simulink model "SWC_FDC_type"  (R2021b)
settings: Solver=FixedStepDiscrete  StartTime=0.0  StopTime=10.0  FixedStep=0.001  RelTol=1e-3
values from neighbouring files (symbols this model uses):
  C_TASK_5MS_S = (	C_TICK_TIME_S      	)    [vcu_local_hdr.m]
  DID_VCUKey = uint16(0x0202)    [vcu_local_hdr.m]
  DID_XWD = uint16(513)    [vcu_local_hdr.m]
  DIDLen_DKCKey = uint16(8)    [vcu_local_hdr.m]
  DIDLen_FoxPiBattSta = uint16(4)    [vcu_local_hdr.m]
  DIDLen_FoxPiBrakeSta = uint16(13)    [vcu_local_hdr.m]
  DIDLen_FoxPiButtonSta = uint16(2)    [vcu_local_hdr.m]
  DIDLen_FoxPiCtrlEnSw = uint16(1)    [vcu_local_hdr.m]
  DIDLen_FoxPiDrivingCtrl = uint16(21)    [vcu_local_hdr.m]
  DIDLen_FoxPiEPSSta = uint16(11)    [vcu_local_hdr.m]
  DIDLen_FoxPiLampCtrl = uint16(6)    [vcu_local_hdr.m]
  DIDLen_FoxPiLampSta = uint16(2)    [vcu_local_hdr.m]
  DIDLen_FoxPiMotionSta = uint16(13)    [vcu_local_hdr.m]
  DIDLen_FoxPiMotorSta = uint16(11)    [vcu_local_hdr.m]
  DIDLen_FoxPiPedalPos = uint16(3)    [vcu_local_hdr.m]
  DIDLen_FoxPiPTGUSSSw = uint16(1)    [vcu_local_hdr.m]
  DIDLen_FoxPiShifterAllow = uint16(3)    [vcu_local_hdr.m]
  DIDLen_FoxPiSwSta = uint16(2)    [vcu_local_hdr.m]
  DIDLen_FoxPiTPMSSta = uint16(13)    [vcu_local_hdr.m]
  DIDLen_FoxPiUSSDist = uint16(20)    [vcu_local_hdr.m]
  DIDLen_FoxPiUSSFaultSta = uint16(2)    [vcu_local_hdr.m]
  DIDLen_FoxPiWheelSpd = uint16(16)    [vcu_local_hdr.m]
  DIDNum_DKCKey = uint16(0x0202)    [vcu_local_hdr.m]
  DIDNum_FoxPiBattSta = uint16(0x100D)    [vcu_local_hdr.m]
  DIDNum_FoxPiBrakeSta = uint16(0x1003)    [vcu_local_hdr.m]
  DIDNum_FoxPiButtonSta = uint16(0x1006)    [vcu_local_hdr.m]
  DIDNum_FoxPiCtrlEnSw = uint16(0x1012)    [vcu_local_hdr.m]
  DIDNum_FoxPiDrivingCtrl = uint16(0x1001)    [vcu_local_hdr.m]
  DIDNum_FoxPiEPSSta = uint16(0x1005)    [vcu_local_hdr.m]
  DIDNum_FoxPiLampCtrl = uint16(0x100C)    [vcu_local_hdr.m]
  DIDNum_FoxPiLampSta = uint16(0x100B)    [vcu_local_hdr.m]
  DIDNum_FoxPiMotionSta = uint16(0x1002)    [vcu_local_hdr.m]
  DIDNum_FoxPiMotorSta = uint16(0x1010)    [vcu_local_hdr.m]
  DIDNum_FoxPiPedalPos = uint16(0x100F)    [vcu_local_hdr.m]
  DIDNum_FoxPiPTGUSSSw = uint16(0x1009)    [vcu_local_hdr.m]
  DIDNum_FoxPiShifterAllow = uint16(0x1011)    [vcu_local_hdr.m]
  DIDNum_FoxPiSwSta = uint16(0x100A)    [vcu_local_hdr.m]
  DIDNum_FoxPiTPMSSta = uint16(0x100E)    [vcu_local_hdr.m]
  DIDNum_FoxPiUSSDist = uint16(0x1007)    [vcu_local_hdr.m]
  DIDNum_FoxPiUSSFaultSta = uint16(0x1008)    [vcu_local_hdr.m]
  DIDNum_FoxPiWheelSpd = uint16(0x1004)    [vcu_local_hdr.m]
  DIDVCUKeyLength = uint16(8)    [vcu_local_hdr.m]
  DTC_10020B = Simulink.Parameter    [DTC_Constant_Definition.m]
  DTC_10020C = Simulink.Parameter    [DTC_Constant_Definition.m]
  DTC_10020D = Simulink.Parameter    [DTC_Constant_Definition.m]
  DTC_10020E = Simulink.Parameter    [DTC_Constant_Definition.m]
  DTC_100210 = Simulink.Parameter    [DTC_Constant_Definition.m]
  DTC_100211 = Simulink.Parameter    [DTC_Constant_Definition.m]
  DTC_100212 = Simulink.Parameter    [DTC_Constant_Definition.m]
  DTC_100213 = Simulink.Parameter    [DTC_Constant_Definition.m]
  DTC_100214 = Simulink.Parameter    [DTC_Constant_Definition.m]
  DTC_100215 = Simulink.Parameter    [DTC_Constant_Definition.m]
  DTC_100216 = Simulink.Parameter    [DTC_Constant_Definition.m]
  DTC_100217 = Simulink.Parameter    [DTC_Constant_Definition.m]
  DTC_100218 = Simulink.Parameter    [DTC_Constant_Definition.m]
  DTC_100219 = Simulink.Parameter    [DTC_Constant_Definition.m]
  DTC_10021A = Simulink.Parameter    [DTC_Constant_Definition.m]
  DTC_10021B = Simulink.Parameter    [DTC_Constant_Definition.m]
  DTC_10021C = Simulink.Parameter    [DTC_Constant_Definition.m]
  DTC_10021D = Simulink.Parameter    [DTC_Constant_Definition.m]
  DTC_10021E = Simulink.Parameter    [DTC_Constant_Definition.m]
  DTC_100220 = Simulink.Parameter    [DTC_Constant_Definition.m]
  DTC_100221 = Simulink.Parameter    [DTC_Constant_Definition.m]
  DTC_100223 = Simulink.Parameter    [DTC_Constant_Definition.m]
  DTC_100224 = Simulink.Parameter    [DTC_Constant_Definition.m]
  DTC_100225 = Simulink.Parameter    [DTC_Constant_Definition.m]
  DTC_100226 = Simulink.Parameter    [DTC_Constant_Definition.m]
  DTC_100227 = Simulink.Parameter    [DTC_Constant_Definition.m]
  DTC_100242 = Simulink.Parameter    [DTC_Constant_Definition.m]
  DTC_100243 = Simulink.Parameter    [DTC_Constant_Definition.m]
  DTC_100244 = Simulink.Parameter    [DTC_Constant_Definition.m]
  DTC_100247 = Simulink.Parameter    [DTC_Constant_Definition.m]
  DTC_100248 = Simulink.Parameter    [DTC_Constant_Definition.m]
  DTC_100249 = Simulink.Parameter    [DTC_Constant_Definition.m]
  DTC_100250 = Simulink.Parameter    [DTC_Constant_Definition.m]
  DTC_100251 = Simulink.Parameter    [DTC_Constant_Definition.m]
  DTC_100252 = Simulink.Parameter    [DTC_Constant_Definition.m]
  DTC_100A10 = Simulink.Parameter    [DTC_Constant_Definition.m]
  DTC_100A12 = Simulink.Parameter    [DTC_Constant_Definition.m]
  DTC_100A16 = Simulink.Parameter    [DTC_Constant_Definition.m]
  DTC_100A17 = Simulink.Parameter    [DTC_Constant_Definition.m]
  DTC_100A18 = Simulink.Parameter    [DTC_Constant_Definition.m]
  DTC_100A19 = Simulink.Parameter    [DTC_Constant_Definition.m]
  DTC_500B01 = Simulink.Parameter    [DTC_Constant_Definition.m]
  DTC_500B02 = Simulink.Parameter    [DTC_Constant_Definition.m]
  DTC_500B03 = Simulink.Parameter    [DTC_Constant_Definition.m]
  DTC_500B04 = Simulink.Parameter    [DTC_Constant_Definition.m]
  DTC_500B05 = Simulink.Parameter    [DTC_Constant_Definition.m]
  DTC_500B06 = Simulink.Parameter    [DTC_Constant_Definition.m]
  DTC_500B07 = Simulink.Parameter    [DTC_Constant_Definition.m]
  DTC_500B08 = Simulink.Parameter    [DTC_Constant_Definition.m]
  DTC_500B09 = Simulink.Parameter    [DTC_Constant_Definition.m]
  DTC_500B0A = Simulink.Parameter    [DTC_Constant_Definition.m]
  DTC_500B0B = Simulink.Parameter    [DTC_Constant_Definition.m]
  DTC_500B0C = Simulink.Parameter    [DTC_Constant_Definition.m]
  DTC_500B0D = Simulink.Parameter    [DTC_Constant_Definition.m]
  DTC_500B0E = Simulink.Parameter    [DTC_Constant_Definition.m]
  DTC_500B0F = Simulink.Parameter    [DTC_Constant_Definition.m]
  DTC_500B10 = Simulink.Parameter    [DTC_Constant_Definition.m]
  DTC_90021F = Simulink.Parameter    [DTC_Constant_Definition.m]
  DTC_90022F = Simulink.Parameter    [DTC_Constant_Definition.m]
  DTC_900253 = Simulink.Parameter    [DTC_Constant_Definition.m]
  DTC_900254 = Simulink.Parameter    [DTC_Constant_Definition.m]
  DTC_900301 = Simulink.Parameter    [DTC_Constant_Definition.m]
  DTC_900302 = Simulink.Parameter    [DTC_Constant_Definition.m]
  DTC_900303 = Simulink.Parameter    [DTC_Constant_Definition.m]
  DTC_900304 = Simulink.Parameter    [DTC_Constant_Definition.m]
  DTC_900305 = Simulink.Parameter    [DTC_Constant_Definition.m]
  DTC_900909 = Simulink.Parameter    [DTC_Constant_Definition.m]
  DTC_90090A = Simulink.Parameter    [DTC_Constant_Definition.m]
  DTC_90090B = Simulink.Parameter    [DTC_Constant_Definition.m]
  DTC_90090C = Simulink.Parameter    [DTC_Constant_Definition.m]
  DTC_90090D = Simulink.Parameter    [DTC_Constant_Definition.m]
  DTC_90090E = Simulink.Parameter    [DTC_Constant_Definition.m]
  DTC_90090F = Simulink.Parameter    [DTC_Constant_Definition.m]
  DTC_900910 = Simulink.Parameter    [DTC_Constant_Definition.m]
  DTC_900911 = Simulink.Parameter    [DTC_Constant_Definition.m]
  DTC_900912 = Simulink.Parameter    [DTC_Constant_Definition.m]
  DTC_900913 = Simulink.Parameter    [DTC_Constant_Definition.m]
  DTC_900914 = Simulink.Parameter    [DTC_Constant_Definition.m]
  ... (+54 more)
undefined symbols (not defined in the file or in its folder): f32_ApsOutVehSpdSig, KHAL_CANBusOffDebounce_cnt, KHAL_CANBusOffDebounce_s, KHAL_DKCDecryptEnable_flg_ovrdflg, KHAL_DKCDecryptEnable_flg_ovrdval, KHAL_RandomNumberY1_enum, KHAL_RandomNumberY2_enum, KHAL_RandomNumberY_ovrdflg, KHAL_TPMSRESBUTT_flg_ovrdflg, KHAL_TPMSRESBUTT_flg_ovrdval, KINP_ReadVinCode_flg, P_boolean, R_DIDWriteCDD_CSOP_DIDSet_DKCKey, R_DIDWriteCDD_CSOP_DIDSet_FoxPiBattSta, R_DIDWriteCDD_CSOP_DIDSet_FoxPiBrakeSta, R_DIDWriteCDD_CSOP_DIDSet_FoxPiButtonSta, R_DIDWriteCDD_CSOP_DIDSet_FoxPiCtrlEnSw, R_DIDWriteCDD_CSOP_DIDSet_FoxPiDrivingCtrl, R_DIDWriteCDD_CSOP_DIDSet_FoxPiEPSSta, R_DIDWriteCDD_CSOP_DIDSet_FoxPiLampCtrl, R_DIDWriteCDD_CSOP_DIDSet_FoxPiLampSta, R_DIDWriteCDD_CSOP_DIDSet_FoxPiMotionSta, R_DIDWriteCDD_CSOP_DIDSet_FoxPiMotorSta, R_DIDWriteCDD_CSOP_DIDSet_FoxPiPedalPos, R_DIDWriteCDD_CSOP_DIDSet_FoxPiPTGUSSSw, R_DIDWriteCDD_CSOP_DIDSet_FoxPiShifterAllow, R_DIDWriteCDD_CSOP_DIDSet_FoxPiSwSta, R_DIDWriteCDD_CSOP_DIDSet_FoxPiTPMSSta, R_DIDWriteCDD_CSOP_DIDSet_FoxPiUSSDist, R_DIDWriteCDD_CSOP_DIDSet_FoxPiUSSFaultSta, R_DIDWriteCDD_CSOP_DIDSet_FoxPiWheelSpd, R_E2E_CAN3_VCU1_CSOP_Write_CAN3_VCU1, R_E2E_CAN3_VCU1_toNIDEC_CSOP_Write_CAN3_VCU1_toNIDEC, R_E2E_CAN4_VCU1_CSOP_Write_CAN4_VCU1, R_FDCCDD_Inner_CSOP_FDC_AppCallSleep, R_HALIN_IMU_CSOP_IMUSetSta, R_HALINCDD_CSOP_PAS_Handler, R_HALINCDD_CSOP_ResetPedalZeroPosDone, R_HALINCDD_CSOP_TPMSSensorIDRegSetResults, R_HALINCDD_CSOP_UDS_Main, R_HALOUT_APS_CSOP_ApsOutput, R_HALOUTCDD_CSOP_AppNmStateReq, R_HALOUTCDD_CSOP_IVIReset, R_HALOUTCDD_CSOP_SetAcoreRebootCmdACK, R_HALOUTCDD_CSOP_SetSysPwrStat ... (+80)
libraries: FVT_lib x447, simulink x289, hcu_lib x19, hdlsllib x9, app x1, halin x1, halout x1, matrix_library x1, inp x1, outp x1
(part 12 of 15)

== system SWC_FDC_type/run_SWC_FDC_RxTx_5ms_sys/Halin_CDD/Halin_SYS/FlashMFSWTri_Verify ==
  In1 : Inport
  Compare To Constant : simulink/Logic and Bit Operations/Compare To Constant  relop=>  const=1  OutDataTypeStr=boolean
  Compare To Constant1 : simulink/Logic and Bit Operations/Compare To Constant  relop=<  const=0  OutDataTypeStr=boolean
  Constant : Constant  Value=ZERO_INT
  Logical Operator : Logic  Operator=OR  AllPortsSameDT=off  OutDataTypeStr=boolean
  Switch : Switch  Criteria=u2 > Threshold
  Out1 : Outport
  wires:
  Compare To Constant1/1 -> Logical Operator/2
  Compare To Constant/1 -> Logical Operator/1
  Logical Operator/1 -> Switch/2
  Switch/1 -> Out1/1
  Constant/1 -> Switch/1
  In1/1 -> Compare To Constant/1, Compare To Constant1/1, Switch/3

== system SWC_FDC_type/run_SWC_FDC_RxTx_5ms_sys/Halin_CDD/Halin_SYS/FlashMirrorFlodPos_Verify ==
  In1 : Inport
  Compare To Constant : simulink/Logic and Bit Operations/Compare To Constant  relop=>  const=1  OutDataTypeStr=boolean
  Compare To Constant1 : simulink/Logic and Bit Operations/Compare To Constant  relop=<  const=0  OutDataTypeStr=boolean
  Constant : Constant  Value=ZERO_INT
  Logical Operator : Logic  Operator=OR  AllPortsSameDT=off  OutDataTypeStr=boolean
  Switch : Switch  Criteria=u2 > Threshold
  Out1 : Outport
  wires:
  In1/1 -> Switch/3, Compare To Constant1/1, Compare To Constant/1
  Constant/1 -> Switch/1
  Switch/1 -> Out1/1
  Logical Operator/1 -> Switch/2
  Compare To Constant/1 -> Logical Operator/1
  Compare To Constant1/1 -> Logical Operator/2

== system SWC_FDC_type/run_SWC_FDC_RxTx_5ms_sys/Halin_CDD/Halin_SYS/FlashRecAutoFlg_Verify ==
  In1 : Inport
  Compare To Constant : simulink/Logic and Bit Operations/Compare To Constant  relop=>  const=1  OutDataTypeStr=boolean
  Compare To Constant1 : simulink/Logic and Bit Operations/Compare To Constant  relop=<  const=0  OutDataTypeStr=boolean
  Constant : Constant  Value=ZERO_INT
  Logical Operator : Logic  Operator=OR  AllPortsSameDT=off  OutDataTypeStr=boolean
  Switch : Switch  Criteria=u2 > Threshold
  Out1 : Outport
  wires:
  In1/1 -> Switch/3, Compare To Constant1/1, Compare To Constant/1
  Constant/1 -> Switch/1
  Switch/1 -> Out1/1
  Logical Operator/1 -> Switch/2
  Compare To Constant/1 -> Logical Operator/1
  Compare To Constant1/1 -> Logical Operator/2

== system SWC_FDC_type/run_SWC_FDC_RxTx_5ms_sys/Halin_CDD/Halin_SYS/FlashWiperFixMode_Verify ==
  In1 : Inport
  Compare To Constant : simulink/Logic and Bit Operations/Compare To Constant  relop=>  const=1  OutDataTypeStr=boolean
  Compare To Constant1 : simulink/Logic and Bit Operations/Compare To Constant  relop=<  const=0  OutDataTypeStr=boolean
  Constant : Constant  Value=ZERO_INT
  Logical Operator : Logic  Operator=OR  AllPortsSameDT=off  OutDataTypeStr=boolean
  Switch : Switch  Criteria=u2 > Threshold
  Out1 : Outport
  wires:
  Compare To Constant1/1 -> Logical Operator/2
  Compare To Constant/1 -> Logical Operator/1
  Logical Operator/1 -> Switch/2
  Switch/1 -> Out1/1
  Constant/1 -> Switch/1
  In1/1 -> Compare To Constant/1, Compare To Constant1/1, Switch/3

== system SWC_FDC_type/run_SWC_FDC_RxTx_5ms_sys/Halin_CDD/Halin_SYS/Flashfdefog_Verify ==
  In1 : Inport
  Compare To Constant : simulink/Logic and Bit Operations/Compare To Constant  relop=>  const=1  OutDataTypeStr=boolean
  Compare To Constant1 : simulink/Logic and Bit Operations/Compare To Constant  relop=<  const=0  OutDataTypeStr=boolean
  Constant : Constant  Value=ZERO_INT
  Logical Operator : Logic  Operator=OR  AllPortsSameDT=off  OutDataTypeStr=boolean
  Switch : Switch  Criteria=u2 > Threshold
  Out1 : Outport
  wires:
  In1/1 -> Switch/3, Compare To Constant1/1, Compare To Constant/1
  Constant/1 -> Switch/1
  Switch/1 -> Out1/1
  Logical Operator/1 -> Switch/2
  Compare To Constant/1 -> Logical Operator/1
  Compare To Constant1/1 -> Logical Operator/2

== system SWC_FDC_type/run_SWC_FDC_RxTx_5ms_sys/Halin_CDD/Halin_SYS/FlashsigRecircSt_Verify ==
  In1 : Inport
  Compare To Constant : simulink/Logic and Bit Operations/Compare To Constant  relop=>  const=1  OutDataTypeStr=boolean
  Compare To Constant1 : simulink/Logic and Bit Operations/Compare To Constant  relop=<  const=0  OutDataTypeStr=boolean
  Constant : Constant  Value=ZERO_INT
  Logical Operator : Logic  Operator=OR  AllPortsSameDT=off  OutDataTypeStr=boolean
  Switch : Switch  Criteria=u2 > Threshold
  Out1 : Outport
  wires:
  Compare To Constant1/1 -> Logical Operator/2
  Compare To Constant/1 -> Logical Operator/1
  Logical Operator/1 -> Switch/2
  Switch/1 -> Out1/1
  Constant/1 -> Switch/1
  In1/1 -> Compare To Constant/1, Compare To Constant1/1, Switch/3

== system SWC_FDC_type/run_SWC_FDC_RxTx_5ms_sys/Halin_CDD/Halin_SYS/FlashsigSetTempZon1St_Verify ==
  In1 : Inport
  Compare To Constant : simulink/Logic and Bit Operations/Compare To Constant  relop=>  const=32  OutDataTypeStr=boolean
  Compare To Constant1 : simulink/Logic and Bit Operations/Compare To Constant  relop=<  const=17  OutDataTypeStr=boolean
  Constant : Constant  Value=25
  Logical Operator : Logic  Operator=OR  AllPortsSameDT=off  OutDataTypeStr=boolean
  Switch : Switch  Criteria=u2 > Threshold
  Out1 : Outport
  wires:
  In1/1 -> Switch/3, Compare To Constant1/1, Compare To Constant/1
  Constant/1 -> Switch/1
  Switch/1 -> Out1/1
  Logical Operator/1 -> Switch/2
  Compare To Constant/1 -> Logical Operator/1
  Compare To Constant1/1 -> Logical Operator/2

== system SWC_FDC_type/run_SWC_FDC_RxTx_5ms_sys/Halin_CDD/Halin_SYS/FlashsigSetTempZon2StM_Verify ==
  In1 : Inport
  Compare To Constant : simulink/Logic and Bit Operations/Compare To Constant  relop=>  const=32  OutDataTypeStr=boolean
  Compare To Constant1 : simulink/Logic and Bit Operations/Compare To Constant  relop=<  const=17  OutDataTypeStr=boolean
  Constant : Constant  Value=25
  Logical Operator : Logic  Operator=OR  AllPortsSameDT=off  OutDataTypeStr=boolean
  Switch : Switch  Criteria=u2 > Threshold
  Out1 : Outport
  wires:
  Compare To Constant1/1 -> Logical Operator/2
  Compare To Constant/1 -> Logical Operator/1
  Logical Operator/1 -> Switch/2
  Switch/1 -> Out1/1
  Constant/1 -> Switch/1
  In1/1 -> Compare To Constant/1, Compare To Constant1/1, Switch/3

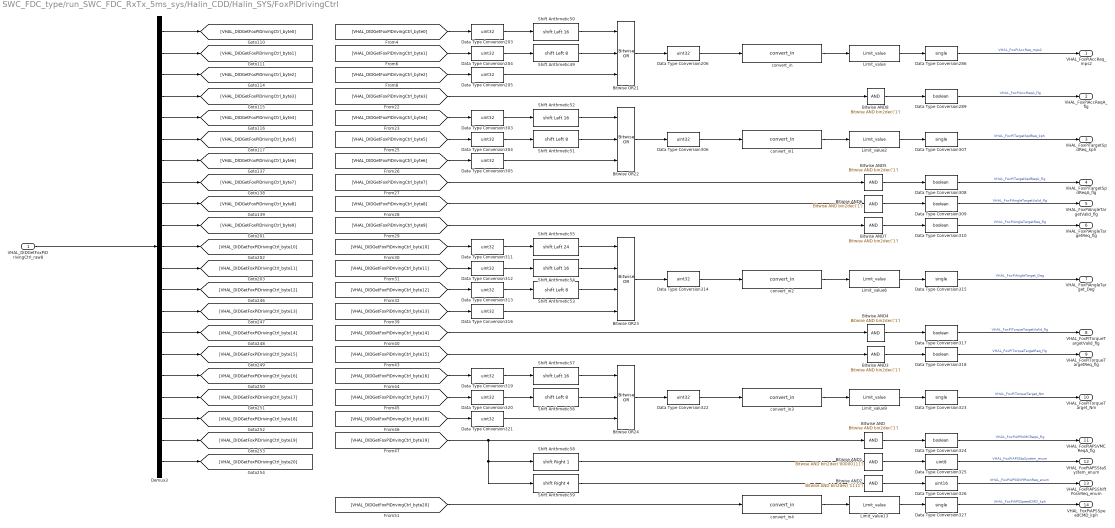
== system SWC_FDC_type/run_SWC_FDC_RxTx_5ms_sys/Halin_CDD/Halin_SYS/FoxPiDrivingCtrl ==
  VHAL_DIDGetFoxPiDrivingCtrl_raw8 : Inport
  Bitwise AND{,3..8} (7 alike) : simulink/Logic and Bit Operations/Bitwise Operator  logicop=AND  UseBitMask=on  BitMask=bin2dec('1')  BitMaskRealWorld=Stored Integer
  Bitwise AND1 : simulink/Logic and Bit Operations/Bitwise Operator  logicop=AND  UseBitMask=on  BitMask=bin2dec('00000111')  BitMaskRealWorld=Stored Integer
  Bitwise AND2 : simulink/Logic and Bit Operations/Bitwise Operator  logicop=AND  UseBitMask=on  BitMask=bin2dec('1111')  BitMaskRealWorld=Stored Integer
  Bitwise OR21 : simulink/Logic and Bit Operations/Bitwise Operator  logicop=OR  UseBitMask=off  NumInputPorts=3  BitMask=bin2dec('00000000000000000000')  BitMaskRealWorld=Stored Integer
  Bitwise OR22 : simulink/Logic and Bit Operations/Bitwise Operator  logicop=OR  UseBitMask=off  NumInputPorts=3  BitMask=bin2dec('00000000000000000000')  BitMaskRealWorld=Stored Integer
  Bitwise OR23 : simulink/Logic and Bit Operations/Bitwise Operator  logicop=OR  UseBitMask=off  NumInputPorts=4  BitMask=bin2dec('00000000000000000000')  BitMaskRealWorld=Stored Integer
  Bitwise OR24 : simulink/Logic and Bit Operations/Bitwise Operator  logicop=OR  UseBitMask=off  NumInputPorts=3  BitMask=bin2dec('00000000000000000000')  BitMaskRealWorld=Stored Integer
  Data Type Conversion{203..206,303..306,311..314,316,319..322} (17 alike) : DataTypeConversion  OutDataTypeStr=uint32
  Data Type Conversion{286,307,315,323,327} (5 alike) : DataTypeConversion  OutDataTypeStr=single
  Data Type Conversion{289,308..310,317..318,324} (7 alike) : DataTypeConversion  OutDataTypeStr=boolean
  Data Type Conversion325 : DataTypeConversion  OutDataTypeStr=uint8
  Data Type Conversion326 : DataTypeConversion  OutDataTypeStr=uint16
  Demux3 : Demux  Outputs=21
  Limit_value : FVT_lib/hal/Limit_value  Upper_limit=10.55  Lower_limit=-15
  Limit_value13 : FVT_lib/hal/Limit_value  Upper_limit=20  Lower_limit=0
  Limit_value2 : FVT_lib/hal/Limit_value  Upper_limit=255.875  Lower_limit=0
  Limit_value6 : FVT_lib/hal/Limit_value  Upper_limit=900  Lower_limit=-900
  Limit_value9 : FVT_lib/hal/Limit_value  Upper_limit=10  Lower_limit=-10
  Shift Arithmetic{49,51,53,56} (4 alike) : ArithShift  BitShiftNumber=8  BitShiftDirection=Left
  Shift Arithmetic{50,52,54,57} (4 alike) : ArithShift  BitShiftNumber=16  BitShiftDirection=Left
  Shift Arithmetic55 : ArithShift  BitShiftNumber=24  BitShiftDirection=Left
  Shift Arithmetic58 : ArithShift  BitShiftNumber=1  BitShiftDirection=Right
  Shift Arithmetic59 : ArithShift  BitShiftNumber=4  BitShiftDirection=Right
  convert_in : FVT_lib/hal/convert_in  gain=0.05  offset=-15
  convert_in1 : FVT_lib/hal/convert_in  gain=0.125  offset=0
  convert_in2 : FVT_lib/hal/convert_in  gain=0.1  offset=-900
  convert_in3 : FVT_lib/hal/convert_in  gain=0.01  offset=-10
  convert_in4 : FVT_lib/hal/convert_in  gain=0.125  offset=0
  VHAL_FoxPiAccReq_mps2 : Outport
  VHAL_FoxPiAccReqA_flg : Outport  Port=2
  VHAL_FoxPiTargetSpdReq_kph : Outport  Port=3
  VHAL_FoxPiTargetSpdReqA_flg : Outport  Port=4
  VHAL_FoxPiAngleTargetValid_flg : Outport  Port=5
  VHAL_FoxPiAngleTargetReq_flg : Outport  Port=6
  VHAL_FoxPiAngleTarget_Deg : Outport  Port=7
  VHAL_FoxPiTorqueTargetValid_flg : Outport  Port=8
  VHAL_FoxPiTorqueTargetReq_flg : Outport  Port=9
  VHAL_FoxPiTorqueTarget_Nm : Outport  Port=10
  VHAL_FoxPiAPSVMCReqA_flg : Outport  Port=11
  VHAL_FoxPiAPSStaSystem_enum : Outport  Port=12
  VHAL_FoxPiAPSShiftPosnReq_enum : Outport  Port=13
  VHAL_FoxPiAPSSpeedCMD_kph : Outport  Port=14
  wires:
  [VHAL_DIDGetFoxPiDrivingCtrl_byte10] -> Data Type Conversion311/1
  [VHAL_DIDGetFoxPiDrivingCtrl_byte20] -> convert_in4/1
  convert_in3/1 -> Limit_value9/1
  [VHAL_DIDGetFoxPiDrivingCtrl_byte14] -> Bitwise AND4/1
  Demux3/14 -> [VHAL_DIDGetFoxPiDrivingCtrl_byte13]
  Data Type Conversion322/1 -> convert_in3/1
  [VHAL_DIDGetFoxPiDrivingCtrl_byte1] -> Data Type Conversion204/1
  [VHAL_DIDGetFoxPiDrivingCtrl_byte19] -> Shift Arithmetic59/1, Shift Arithmetic58/1, Bitwise AND/1
  Data Type Conversion309/1 -> VHAL_FoxPiAngleTargetValid_flg/1  "VHAL_FoxPiAngleTargetValid_flg"
  Data Type Conversion324/1 -> VHAL_FoxPiAPSVMCReqA_flg/1  "VHAL_FoxPiAPSVMCReqA_flg"
  Demux3/4 -> [VHAL_DIDGetFoxPiDrivingCtrl_byte3]
  [VHAL_DIDGetFoxPiDrivingCtrl_byte7] -> Bitwise AND5/1
  [VHAL_DIDGetFoxPiDrivingCtrl_byte8] -> Bitwise AND6/1
  [VHAL_DIDGetFoxPiDrivingCtrl_byte11] -> Data Type Conversion312/1
  [VHAL_DIDGetFoxPiDrivingCtrl_byte5] -> Data Type Conversion304/1
  Bitwise OR24/1 -> Data Type Conversion322/1
  Data Type Conversion325/1 -> VHAL_FoxPiAPSStaSystem_enum/1  "VHAL_FoxPiAPSStaSystem_enum"
  [VHAL_DIDGetFoxPiDrivingCtrl_byte17] -> Data Type Conversion320/1
  Data Type Conversion314/1 -> convert_in2/1
  [VHAL_DIDGetFoxPiDrivingCtrl_byte16] -> Data Type Conversion319/1
  Bitwise OR22/1 -> Data Type Conversion306/1
  Shift Arithmetic59/1 -> Bitwise AND2/1
  Demux3/2 -> [VHAL_DIDGetFoxPiDrivingCtrl_byte1]
  [VHAL_DIDGetFoxPiDrivingCtrl_byte12] -> Data Type Conversion313/1
  [VHAL_DIDGetFoxPiDrivingCtrl_byte2] -> Data Type Conversion205/1
  Data Type Conversion306/1 -> convert_in1/1
  [VHAL_DIDGetFoxPiDrivingCtrl_byte4] -> Data Type Conversion303/1
  Data Type Conversion307/1 -> VHAL_FoxPiTargetSpdReq_kph/1  "VHAL_FoxPiTargetSpdReq_kph"
  Data Type Conversion326/1 -> VHAL_FoxPiAPSShiftPosnReq_enum/1  "VHAL_FoxPiAPSShiftPosnReq_enum"
  Data Type Conversion304/1 -> Shift Arithmetic51/1
  Demux3/1 -> [VHAL_DIDGetFoxPiDrivingCtrl_byte0]
  convert_in4/1 -> Limit_value13/1
  Data Type Conversion323/1 -> VHAL_FoxPiTorqueTarget_Nm/1  "VHAL_FoxPiTorqueTarget_Nm"
  [VHAL_DIDGetFoxPiDrivingCtrl_byte9] -> Bitwise AND7/1
  [VHAL_DIDGetFoxPiDrivingCtrl_byte13] -> Data Type Conversion316/1
  Demux3/11 -> [VHAL_DIDGetFoxPiDrivingCtrl_byte10]
  Bitwise OR21/1 -> Data Type Conversion206/1
  convert_in2/1 -> Limit_value6/1
  [VHAL_DIDGetFoxPiDrivingCtrl_byte18] -> Data Type Conversion321/1
  Demux3/3 -> [VHAL_DIDGetFoxPiDrivingCtrl_byte2]
  Bitwise OR23/1 -> Data Type Conversion314/1
  Data Type Conversion206/1 -> convert_in/1
  [VHAL_DIDGetFoxPiDrivingCtrl_byte6] -> Data Type Conversion305/1
  [VHAL_DIDGetFoxPiDrivingCtrl_byte15] -> Bitwise AND3/1
  convert_in1/1 -> Limit_value2/1
  [VHAL_DIDGetFoxPiDrivingCtrl_byte0] -> Data Type Conversion203/1
  Shift Arithmetic58/1 -> Bitwise AND1/1
  Demux3/7 -> [VHAL_DIDGetFoxPiDrivingCtrl_byte6]
  Demux3/8 -> [VHAL_DIDGetFoxPiDrivingCtrl_byte7]
  Demux3/5 -> [VHAL_DIDGetFoxPiDrivingCtrl_byte4]
  Demux3/6 -> [VHAL_DIDGetFoxPiDrivingCtrl_byte5]
  Demux3/10 -> [VHAL_DIDGetFoxPiDrivingCtrl_byte9]
  Demux3/12 -> [VHAL_DIDGetFoxPiDrivingCtrl_byte11]
  Demux3/9 -> [VHAL_DIDGetFoxPiDrivingCtrl_byte8]
  Demux3/13 -> [VHAL_DIDGetFoxPiDrivingCtrl_byte12]
  Demux3/21 -> [VHAL_DIDGetFoxPiDrivingCtrl_byte20]
  Demux3/15 -> [VHAL_DIDGetFoxPiDrivingCtrl_byte14]
  Demux3/16 -> [VHAL_DIDGetFoxPiDrivingCtrl_byte15]
  Data Type Conversion317/1 -> VHAL_FoxPiTorqueTargetValid_flg/1  "VHAL_FoxPiTorqueTargetValid_flg"
  Demux3/17 -> [VHAL_DIDGetFoxPiDrivingCtrl_byte16]
  Demux3/20 -> [VHAL_DIDGetFoxPiDrivingCtrl_byte19]
  Demux3/18 -> [VHAL_DIDGetFoxPiDrivingCtrl_byte17]
  Demux3/19 -> [VHAL_DIDGetFoxPiDrivingCtrl_byte18]
  Data Type Conversion289/1 -> VHAL_FoxPiAccReqA_flg/1  "VHAL_FoxPiAccReqA_flg"
  Data Type Conversion315/1 -> VHAL_FoxPiAngleTarget_Deg/1  "VHAL_FoxPiAngleTarget_Deg"
  Data Type Conversion327/1 -> VHAL_FoxPiAPSSpeedCMD_kph/1  "VHAL_FoxPiAPSSpeedCMD_kph"
  Data Type Conversion310/1 -> VHAL_FoxPiAngleTargetReq_flg/1  "VHAL_FoxPiAngleTargetReq_flg"
  Data Type Conversion308/1 -> VHAL_FoxPiTargetSpdReqA_flg/1  "VHAL_FoxPiTargetSpdReqA_flg"
  Data Type Conversion286/1 -> VHAL_FoxPiAccReq_mps2/1  "VHAL_FoxPiAccReq_mps2"
  Data Type Conversion318/1 -> VHAL_FoxPiTorqueTargetReq_flg/1  "VHAL_FoxPiTorqueTargetReq_flg"
  VHAL_DIDGetFoxPiDrivingCtrl_raw8/1 -> Demux3/1
  Data Type Conversion319/1 -> Shift Arithmetic57/1
  Data Type Conversion320/1 -> Shift Arithmetic56/1
  Shift Arithmetic57/1 -> Bitwise OR24/1
  Shift Arithmetic56/1 -> Bitwise OR24/2
  Data Type Conversion321/1 -> Bitwise OR24/3
  Data Type Conversion311/1 -> Shift Arithmetic55/1
  Data Type Conversion312/1 -> Shift Arithmetic54/1
  Data Type Conversion313/1 -> Shift Arithmetic53/1
  Shift Arithmetic55/1 -> Bitwise OR23/1
  Shift Arithmetic54/1 -> Bitwise OR23/2
  Shift Arithmetic53/1 -> Bitwise OR23/3
  Data Type Conversion316/1 -> Bitwise OR23/4
  Data Type Conversion303/1 -> Shift Arithmetic52/1
  Shift Arithmetic52/1 -> Bitwise OR22/1
  Shift Arithmetic51/1 -> Bitwise OR22/2
  Data Type Conversion305/1 -> Bitwise OR22/3
  Data Type Conversion203/1 -> Shift Arithmetic50/1
  Data Type Conversion204/1 -> Shift Arithmetic49/1
  Shift Arithmetic50/1 -> Bitwise OR21/1
  Shift Arithmetic49/1 -> Bitwise OR21/2
  Data Type Conversion205/1 -> Bitwise OR21/3
  convert_in/1 -> Limit_value/1
  Limit_value/1 -> Data Type Conversion286/1
  [VHAL_DIDGetFoxPiDrivingCtrl_byte3] -> Bitwise AND8/1
  Limit_value2/1 -> Data Type Conversion307/1
  Limit_value6/1 -> Data Type Conversion315/1
  Bitwise AND4/1 -> Data Type Conversion317/1
  Bitwise AND3/1 -> Data Type Conversion318/1
  Limit_value9/1 -> Data Type Conversion323/1
  Bitwise AND/1 -> Data Type Conversion324/1
  Bitwise AND1/1 -> Data Type Conversion325/1
  Bitwise AND2/1 -> Data Type Conversion326/1
  Limit_value13/1 -> Data Type Conversion327/1
  Bitwise AND5/1 -> Data Type Conversion308/1
  Bitwise AND6/1 -> Data Type Conversion309/1
  Bitwise AND7/1 -> Data Type Conversion310/1
  Bitwise AND8/1 -> Data Type Conversion289/1

== system SWC_FDC_type/run_SWC_FDC_RxTx_5ms_sys/Halin_CDD/Halin_SYS/Subsystem ==
  VHAL_DIDGetFoxPiLampCtrl_raw8 : Inport
  Bitwise AND{1..21} (21 alike) : simulink/Logic and Bit Operations/Bitwise Operator  logicop=AND  UseBitMask=on  BitMask=bin2dec('1')  BitMaskRealWorld=Stored Integer
  Bitwise AND22 : simulink/Logic and Bit Operations/Bitwise Operator  logicop=AND  UseBitMask=on  BitMask=bin2dec('111')  BitMaskRealWorld=Stored Integer
  Data Type Conversion{203..206,286,289,303..314,316..317,324} (21 alike) : DataTypeConversion  OutDataTypeStr=boolean
  Data Type Conversion{315,319..321} (4 alike) : DataTypeConversion  OutDataTypeStr=uint8
  Demux3 : Demux  Outputs=6
  Limit_value1 : FVT_lib/hal/Limit_value  Upper_limit=7  Lower_limit=0
  Limit_value2 : FVT_lib/hal/Limit_value  Upper_limit=100  Lower_limit=0
  Limit_value3 : FVT_lib/hal/Limit_value  Upper_limit=63  Lower_limit=0
  Shift Arithmetic49 : ArithShift  BitShiftNumber=2  BitShiftDirection=Right
  Shift Arithmetic50 : ArithShift  BitShiftNumber=4  BitShiftDirection=Right
  Shift Arithmetic51 : ArithShift  BitShiftNumber=3  BitShiftDirection=Right
  Shift Arithmetic52 : ArithShift  BitShiftNumber=5  BitShiftDirection=Right
  Shift Arithmetic53 : ArithShift  BitShiftNumber=7  BitShiftDirection=Right
  Shift Arithmetic54 : ArithShift  BitShiftNumber=6  BitShiftDirection=Right
  Shift Arithmetic55 : ArithShift  BitShiftNumber=2  BitShiftDirection=Right
  Shift Arithmetic56 : ArithShift  BitShiftNumber=4  BitShiftDirection=Right
  Shift Arithmetic57 : ArithShift  BitShiftNumber=3  BitShiftDirection=Right
  Shift Arithmetic58 : ArithShift  BitShiftNumber=1  BitShiftDirection=Right
  Shift Arithmetic59 : ArithShift  BitShiftNumber=5  BitShiftDirection=Right
  Shift Arithmetic60 : ArithShift  BitShiftNumber=7  BitShiftDirection=Right
  Shift Arithmetic61 : ArithShift  BitShiftNumber=6  BitShiftDirection=Right
  Shift Arithmetic62 : ArithShift  BitShiftNumber=1  BitShiftDirection=Right
  Shift Arithmetic63 : ArithShift  BitShiftNumber=2  BitShiftDirection=Right
  Shift Arithmetic64 : ArithShift  BitShiftNumber=4  BitShiftDirection=Right
  Shift Arithmetic65 : ArithShift  BitShiftNumber=3  BitShiftDirection=Right
  Shift Arithmetic66 : ArithShift  BitShiftNumber=5  BitShiftDirection=Right
  Shift Arithmetic67 : ArithShift  BitShiftNumber=1  BitShiftDirection=Right
  VHAL_FoxPiPosLampCtrlEN_flg : Outport
  VHAL_FoxPiPosLampCtrl_flg : Outport  Port=2
  VHAL_FoxPiLBeamCtrlEN_flg : Outport  Port=3
  VHAL_FoxPiLBeamCtrl_flg : Outport  Port=4
  VHAL_FoxPiHBeamCtrlEN_flg : Outport  Port=5
  VHAL_FoxPiHBeamCtrl_flg : Outport  Port=6
  VHAL_FoxPiRDRLCtrlEN_flg : Outport  Port=7
  VHAL_FoxPiRDRLCtrl_flg : Outport  Port=8
  VHAL_FoxPiLDRLCtrlEN_flg : Outport  Port=9
  VHAL_FoxPiLDRLCtrl_flg : Outport  Port=10
  VHAL_FoxPiLTurnLPCtrlEN_flg : Outport  Port=11
  VHAL_FoxPiLTurnLPCtrl_flg : Outport  Port=12
  VHAL_FoxPiRTurnLPCtrlEN_flg : Outport  Port=13
  VHAL_FoxPiRTurnLPCtrl_flg : Outport  Port=14
  VHAL_FoxPiBkLampCtrlEN_flg : Outport  Port=15
  VHAL_FoxPiBkLampCtrl_flg : Outport  Port=16
  VHAL_FoxPiRevCtrlEN_flg : Outport  Port=17
  VHAL_FoxPiRevCtrl_flg : Outport  Port=18
  VHAL_FoxPiRrFogLpCtrlEN_flg : Outport  Port=19
  VHAL_FoxPiRrFogLpCtrl_flg : Outport  Port=20
  VHAL_FoxPiAmbCtrlEN_flg : Outport  Port=21
  VHAL_FoxPiAmbAreaCtrl_enum : Outport  Port=22
  VHAL_FoxPiAmbColorCtrl_enum : Outport  Port=23
  VHAL_FoxPiAmbBrightCtrl_enum : Outport  Port=24
  VHAL_FoxPiAmbBreathCtrl_enum : Outport  Port=25
  wires:
  Data Type Conversion316/1 -> VHAL_FoxPiRrFogLpCtrl_flg/1  "VHAL_FoxPiRrFogLpCtrl_flg"
  Demux3/1 -> [VHAL_DIDGetFoxPiLampCtrl_byte0]
  Data Type Conversion315/1 -> VHAL_FoxPiAmbAreaCtrl_enum/1  "VHAL_FoxPiAmbAreaCtrl_enum"
  Demux3/3 -> [VHAL_DIDGetFoxPiLampCtrl_byte2]
  [VHAL_DIDGetFoxPiLampCtrl_byte1] -> Bitwise AND12/1, Shift Arithmetic62/1, Shift Arithmetic55/1, Shift Arithmetic57/1, Shift Arithmetic56/1, Shift Arithmetic59/1, Shift Arithmetic61/1, Shift Arithmetic60/1
  Shift Arithmetic49/1 -> Bitwise AND3/1
  Data Type Conversion313/1 -> VHAL_FoxPiRrFogLpCtrlEN_flg/1  "VHAL_FoxPiRrFogLpCtrlEN_flg"
  Demux3/5 -> [VHAL_DIDGetFoxPiLampCtrl_byte4]
  Shift Arithmetic53/1 -> Bitwise AND6/1
  Data Type Conversion203/1 -> VHAL_FoxPiPosLampCtrl_flg/1  "VHAL_FoxPiPosLampCtrl_flg"
  Data Type Conversion289/1 -> VHAL_FoxPiRDRLCtrlEN_flg/1  "VHAL_FoxPiRDRLCtrlEN_flg"
  [VHAL_DIDGetFoxPiLampCtrl_byte2] -> Shift Arithmetic66/1, Shift Arithmetic64/1, Shift Arithmetic65/1, Shift Arithmetic63/1, Shift Arithmetic67/1, Bitwise AND17/1
  Shift Arithmetic50/1 -> Bitwise AND8/1
  Data Type Conversion307/1 -> VHAL_FoxPiRTurnLPCtrl_flg/1  "VHAL_FoxPiRTurnLPCtrl_flg"
  Shift Arithmetic59/1 -> Bitwise AND13/1
  Shift Arithmetic55/1 -> Bitwise AND11/1
  [VHAL_DIDGetFoxPiLampCtrl_byte0] -> Shift Arithmetic53/1, Shift Arithmetic54/1, Shift Arithmetic52/1, Shift Arithmetic50/1, Shift Arithmetic51/1, Shift Arithmetic49/1, Shift Arithmetic58/1, Bitwise AND4/1
  Shift Arithmetic64/1 -> Bitwise AND19/1
  Data Type Conversion309/1 -> VHAL_FoxPiBkLampCtrlEN_flg/1  "VHAL_FoxPiBkLampCtrlEN_flg"
  Data Type Conversion319/1 -> VHAL_FoxPiAmbColorCtrl_enum/1  "VHAL_FoxPiAmbColorCtrl_enum"
  Shift Arithmetic67/1 -> Bitwise AND21/1
  Data Type Conversion286/1 -> VHAL_FoxPiLBeamCtrl_flg/1  "VHAL_FoxPiLBeamCtrl_flg"
  [VHAL_DIDGetFoxPiLampCtrl_byte4] -> Limit_value2/1
  Shift Arithmetic63/1 -> Bitwise AND18/1
  Data Type Conversion324/1 -> VHAL_FoxPiPosLampCtrlEN_flg/1  "VHAL_FoxPiPosLampCtrlEN_flg"
  Shift Arithmetic65/1 -> Bitwise AND20/1
  Data Type Conversion205/1 -> VHAL_FoxPiHBeamCtrlEN_flg/1  "VHAL_FoxPiHBeamCtrlEN_flg"
  Shift Arithmetic62/1 -> Bitwise AND9/1
  Shift Arithmetic57/1 -> Bitwise AND10/1
  Shift Arithmetic66/1 -> Bitwise AND22/1
  Demux3/2 -> [VHAL_DIDGetFoxPiLampCtrl_byte1]
  Shift Arithmetic56/1 -> Bitwise AND16/1
  Shift Arithmetic54/1 -> Bitwise AND7/1
  Demux3/6 -> [VHAL_DIDGetFoxPiLampCtrl_byte5]
  Data Type Conversion317/1 -> VHAL_FoxPiRevCtrlEN_flg/1  "VHAL_FoxPiRevCtrlEN_flg"
  Shift Arithmetic60/1 -> Bitwise AND14/1
  Shift Arithmetic52/1 -> Bitwise AND5/1
  Data Type Conversion305/1 -> VHAL_FoxPiLTurnLPCtrlEN_flg/1  "VHAL_FoxPiLTurnLPCtrlEN_flg"
  Shift Arithmetic58/1 -> Bitwise AND1/1
  Demux3/4 -> [VHAL_DIDGetFoxPiLampCtrl_byte3]
  Shift Arithmetic61/1 -> Bitwise AND15/1
  Data Type Conversion311/1 -> VHAL_FoxPiLDRLCtrlEN_flg/1  "VHAL_FoxPiLDRLCtrlEN_flg"
  Shift Arithmetic51/1 -> Bitwise AND2/1
  [VHAL_DIDGetFoxPiLampCtrl_byte3] -> Limit_value3/1
  Data Type Conversion204/1 -> VHAL_FoxPiLBeamCtrlEN_flg/1  "VHAL_FoxPiLBeamCtrlEN_flg"
  VHAL_DIDGetFoxPiLampCtrl_raw8/1 -> Demux3/1
  Data Type Conversion304/1 -> VHAL_FoxPiLDRLCtrl_flg/1  "VHAL_FoxPiLDRLCtrl_flg"
  Data Type Conversion310/1 -> VHAL_FoxPiBkLampCtrl_flg/1  "VHAL_FoxPiBkLampCtrl_flg"
  Data Type Conversion312/1 -> VHAL_FoxPiRevCtrl_flg/1  "VHAL_FoxPiRevCtrl_flg"
  Data Type Conversion308/1 -> VHAL_FoxPiLTurnLPCtrl_flg/1  "VHAL_FoxPiLTurnLPCtrl_flg"
  Data Type Conversion314/1 -> VHAL_FoxPiAmbCtrlEN_flg/1  "VHAL_FoxPiAmbCtrlEN_flg"
  Data Type Conversion320/1 -> VHAL_FoxPiAmbBrightCtrl_enum/1  "VHAL_FoxPiAmbBrightCtrl_enum"
  Data Type Conversion303/1 -> VHAL_FoxPiRDRLCtrl_flg/1  "VHAL_FoxPiRDRLCtrl_flg"
  Data Type Conversion206/1 -> VHAL_FoxPiHBeamCtrl_flg/1  "VHAL_FoxPiHBeamCtrl_flg"
  Data Type Conversion306/1 -> VHAL_FoxPiRTurnLPCtrlEN_flg/1  "VHAL_FoxPiRTurnLPCtrlEN_flg"
  Data Type Conversion321/1 -> VHAL_FoxPiAmbBreathCtrl_enum/1  "VHAL_FoxPiAmbBreathCtrl_enum"
  Bitwise AND4/1 -> Data Type Conversion324/1
  Bitwise AND1/1 -> Data Type Conversion203/1
  Bitwise AND2/1 -> Data Type Conversion286/1
  Bitwise AND3/1 -> Data Type Conversion204/1
  Bitwise AND5/1 -> Data Type Conversion206/1
  Bitwise AND6/1 -> Data Type Conversion303/1
  Bitwise AND7/1 -> Data Type Conversion289/1
  Bitwise AND8/1 -> Data Type Conversion205/1
  Bitwise AND10/1 -> Data Type Conversion308/1
  Bitwise AND9/1 -> Data Type Conversion304/1
  Bitwise AND11/1 -> Data Type Conversion305/1
  Bitwise AND14/1 -> Data Type Conversion310/1
  Bitwise AND13/1 -> Data Type Conversion307/1
  Bitwise AND15/1 -> Data Type Conversion309/1
  Bitwise AND12/1 -> Data Type Conversion311/1
  Bitwise AND16/1 -> Data Type Conversion306/1
  Bitwise AND17/1 -> Data Type Conversion317/1
  Bitwise AND19/1 -> Data Type Conversion314/1
  Bitwise AND18/1 -> Data Type Conversion313/1
  Bitwise AND20/1 -> Data Type Conversion316/1
  Bitwise AND21/1 -> Data Type Conversion312/1
  Bitwise AND22/1 -> Data Type Conversion315/1
  Limit_value2/1 -> Data Type Conversion320/1
  Limit_value3/1 -> Data Type Conversion319/1
  Limit_value1/1 -> Data Type Conversion321/1
  [VHAL_DIDGetFoxPiLampCtrl_byte5] -> Limit_value1/1

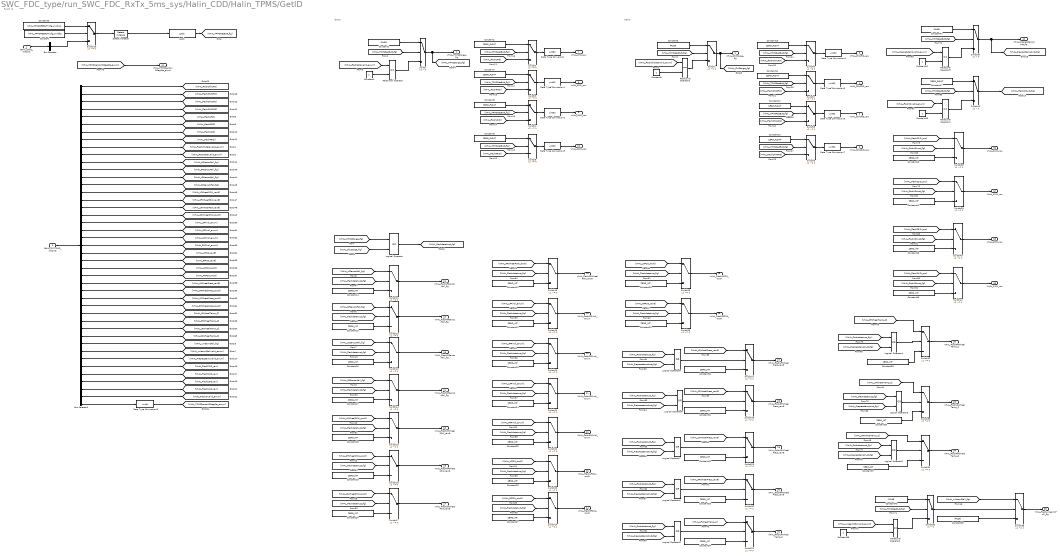
== system SWC_FDC_type/run_SWC_FDC_RxTx_5ms_sys/Halin_CDD/Halin_TPMS/GetID ==
  note: FLASH ID
  note: GetID
  note: GetID
  BHAL_CAN2_outputs : Inport
  BHAL_SYSTPMS_outputs : Inport  Port=2
  Bus Selector : BusSelector  OutputSignals=VHAL_TPMSResButt_flg
  Bus Selector1 : BusSelector  OutputSignals=VHAL_FlashChkLFID_raw,VHAL_FlashChkRFID_raw,VHAL_FlashChkLRID_raw,VHAL_FlashChkRRID_raw,VHAL_FlashLFID_raw,VHAL_FlashRFID_raw,VHAL_FlashLRID_raw,VHAL_FlashRRID_raw,VHAL_Flashchkdatavalid_enum,VHAL_Flashdatavalid_enum,VHAL_LFSensorFail_flg,VHAL_RFSensorFail_flg,VHAL_LRSensorFail_flg,VHAL_RRSensorFail_flg,VHAL_LFWheelPSW_raw8,VHAL_RFWheelPSW_raw8,VHAL_LRWheelPSW_raw8,VHAL_RRWheelPSW_raw8,VHAL_LFPindi_enum,VHAL_RFPindi_enum,VHAL_LRPindi_enum,VHAL_RRPindi_enum,VHAL_LFP20_raw8,VHAL_RFP20_raw8,VHAL_LRP20_raw8,VHAL_RRP20_raw8,VHAL_LFWheelPress_raw8,VHAL_RFWheelPress_raw8,VHAL_LRWheelPress_raw8,VHAL_RRWheelPress_raw8,VHAL_LFWheelTemp_C,VHAL_RFWheelTemp_C,VHAL_LRWheelTemp_C,VHAL_RRWheelTemp_C,VHAL_unlearnSfali_flg,VHAL_unlearnSfailvalid_enum,VHAL_Prepresstempvalid_enum,VHAL_FlashS1ID_raw,VHAL_FlashS2ID_raw,VHAL_FlashS3ID_raw,VHAL_FlashS4ID_raw,VHAL_FlashIDvalid_enum,VHAL_TPMSSensorIDRegSta_raw
  Constant : Constant  Value=KHAL_TPMSRESBUTT_flg_ovrdflg
  Constant{1,7..13,47} (9 alike) : Constant  Value=ZERO_FLOAT
  Constant{14..37,43..46} (28 alike) : Constant  Value=ZERO_INT
  Constant{2..3,38,40..41} (5 alike) : Constant  Value=FALSE
  Constant{4..5,39,42,48} (5 alike) : Constant
  Constant6 : Constant  Value=KHAL_TPMSRESBUTT_flg_ovrdval
  Data Type Conversion{,1..7} (8 alike) : DataTypeConversion  OutDataTypeStr=uint32
  Data Type Conversion8 : DataTypeConversion  OutDataTypeStr=uint8
  Detect Increase : simulink/Logic and Bit Operations/Detect Increase  vinit=0.0  OutDataTypeStr=boolean
  Latch : hcu_lib/Basic_Blocks/Latch
  Logical Operator{,2..9} (9 alike) : Logic  Operator=OR  AllPortsSameDT=off  OutDataTypeStr=boolean
  Relational Operator{,1..4} (5 alike) : RelationalOperator  Operator===  OutDataTypeStr=boolean  RndMeth=Simplest
  Switch{,36..37,42} (4 alike) : Switch  Criteria=u2 > Threshold
  Switch{1..35,38..41} (39 alike) : Switch  Criteria=u2 ~= 0
  VHAL_TPMSStorge_flg : Outport
  VHAL_ChkStorge_flg : Outport  Port=2
  VHAL_ChkLFID_raw : Outport  Port=3
  VHAL_ChkRFID_raw : Outport  Port=4
  VHAL_ChkLRID_raw : Outport  Port=5
  VHAL_ChkRRID_raw : Outport  Port=6
  VHAL_LFID_raw : Outport  Port=7
  VHAL_RFID_raw : Outport  Port=8
  VHAL_LRID_raw : Outport  Port=9
  VHAL_RRID_raw : Outport  Port=10
  VHAL_FlashLFSensorFail_flg : Outport  Port=11
  VHAL_FlashRFSensorFail_flg : Outport  Port=12
  VHAL_FlashLRSensorFail_flg : Outport  Port=13
  VHAL_FlashRRSensorFail_flg : Outport  Port=14
  VHAL_FlashLFWheelPSW_raw8 : Outport  Port=15
  VHAL_FlashRFWheelPSW_raw8 : Outport  Port=16
  VHAL_FlashLRWheelPSW_raw8 : Outport  Port=17
  VHAL_FlashRRWheelPSW_raw8 : Outport  Port=18
  VHAL_FlashLFPindi_enum : Outport  Port=19
  VHAL_FlashRFPindi_enum : Outport  Port=20
  VHAL_FlashLRPindi_enum : Outport  Port=21
  VHAL_FlashRRPindi_enum : Outport  Port=22
  VHAL_FlashLFP20_raw8 : Outport  Port=23
  VHAL_FlashRFP20_raw8 : Outport  Port=24
  VHAL_FlashLRP20_raw8 : Outport  Port=25
  VHAL_FlashRRP20_raw8 : Outport  Port=26
  VHAL_FlashLFWheelPress_raw8 : Outport  Port=27
  VHAL_FlashRFWheelPress_raw8 : Outport  Port=28
  VHAL_FlashLRWheelPress_raw8 : Outport  Port=29
  VHAL_FlashRRWheelPress_raw8 : Outport  Port=30
  VHAL_FlashLFWheelTemp_C : Outport  Port=31
  VHAL_FlashRFWheelTemp_C : Outport  Port=32
  VHAL_FlashLRWheelTemp_C : Outport  Port=33
  VHAL_FlashRRWheelTemp_C : Outport  Port=34
  VHAL_FlashunlearnSfali_flg : Outport  Port=35
  VHAL_S1ID_raw : Outport  Port=36
  VHAL_S2ID_raw : Outport  Port=37
  VHAL_S3ID_raw : Outport  Port=38
  VHAL_S4ID_raw : Outport  Port=39
  VHAL_Prepresstemptrust_flg : Outport  Port=40
  VHAL_TPMSSensorIDRegSta_enum : Outport  Port=41
  wires:
  BHAL_CAN2_outputs/1 -> Bus Selector/1
  Latch/1 -> [VHAL_TPMSResButt_flg]
  [VHAL_TPMSResButt_flg] -> Switch4/2
  [VHAL_TPMSResButt_flg] -> Switch3/2
  [VHAL_FlashChkLFID] -> Switch6/3
  Switch3/1 -> Data Type Conversion1/1
  [VHAL_FlashRFID] -> Switch3/3
  Constant12/1 -> Switch8/1
  Constant9/1 -> Switch5/1
  [VHAL_FlashRRID] -> Switch5/3
  Constant1/1 -> Switch2/1
  Constant7/1 -> Switch3/1
  [VHAL_TPMSResButt_flg] -> Switch9/2
  [VHAL_TPMSResButt_flg] -> Switch2/2
  [VHAL_FlashLRID] -> Switch4/3
  Constant8/1 -> Switch4/1
  Switch2/1 -> Data Type Conversion/1
  [VHAL_TPMSResButt_flg] -> Switch5/2
  Switch4/1 -> Data Type Conversion2/1
  [VHAL_FlashChkLRID] -> Switch8/3
  [VHAL_FlashChkRRID] -> Switch9/3
  Constant10/1 -> Switch6/1
  Constant11/1 -> Switch7/1
  Switch8/1 -> Data Type Conversion6/1
  [VHAL_TPMSResButt_flg] -> Switch6/2
  Switch6/1 -> Data Type Conversion4/1
  Switch9/1 -> Data Type Conversion7/1
  Constant13/1 -> Switch9/1
  Switch7/1 -> Data Type Conversion5/1
  [VHAL_TPMSResButt_flg] -> Switch8/2
  [VHAL_TPMSResButt_flg] -> Switch7/2
  Switch5/1 -> Data Type Conversion3/1
  [VHAL_FlashChkRFID] -> Switch7/3
  [VHAL_FlashLFID] -> Switch2/3
  Switch10/1 -> Detect Increase/1
  Constant/1 -> Switch10/2
  Constant6/1 -> Switch10/1
  Bus Selector/1 -> Switch10/3  "<VHAL_TPMSResButt_flg>"
  [VHAL_TPMSResButt_flg] -> Switch/2
  Switch/1 -> [VHAL_TPMSStorge_flg], VHAL_TPMSStorge_flg/1
  Constant2/1 -> Switch/1
  Constant3/1 -> Switch1/1
  Switch1/1 -> [VHAL_ChkStorge_flg], VHAL_ChkStorge_flg/1
  [VHAL_TPMSResButt_flg] -> Switch1/2
  [VHAL_Flashdatavalid_enum] -> Relational Operator/1
  Relational Operator/1 -> Switch/3
  Constant4/1 -> Relational Operator/2
  Constant5/1 -> Relational Operator1/2
  Relational Operator1/1 -> Switch1/3
  [VHAL_Flashchkdatavalid_enum] -> Relational Operator1/1
  [VHAL_TPMSStorge_flg] -> Logical Operator/1
  [VHAL_ChkStorge_flg] -> Logical Operator/2
  Logical Operator/1 -> [VHAL_Flashdatatrust_flg]
  [VHAL_Flashdatatrust_flg] -> Switch11/2
  [VHAL_LFSensorFail_flg] -> Switch11/1
  Constant14/1 -> Switch11/3
  Switch11/1 -> VHAL_FlashLFSensorFail_flg/1
  Constant15/1 -> Switch12/3
  [VHAL_Flashdatatrust_flg] -> Switch12/2
  Constant16/1 -> Switch13/3
  [VHAL_Flashdatatrust_flg] -> Switch13/2
  Constant17/1 -> Switch14/3
  [VHAL_Flashdatatrust_flg] -> Switch14/2
  Constant18/1 -> Switch15/3
  [VHAL_Flashdatatrust_flg] -> Switch15/2
  Constant19/1 -> Switch16/3
  [VHAL_Flashdatatrust_flg] -> Switch16/2
  Constant20/1 -> Switch17/3
  [VHAL_Flashdatatrust_flg] -> Switch17/2
  Constant21/1 -> Switch18/3
  [VHAL_Flashdatatrust_flg] -> Switch18/2
  [VHAL_RFSensorFail_flg] -> Switch12/1
  [VHAL_LRSensorFail_flg] -> Switch13/1
  [VHAL_RRSensorFail_flg] -> Switch14/1
  [VHAL_LFWheelPSW_raw8] -> Switch15/1
  [VHAL_RFWheelPSW_raw8] -> Switch16/1
  [VHAL_LRWheelPSW_raw8] -> Switch17/1
  [VHAL_RRWheelPSW_raw8] -> Switch18/1
  Constant22/1 -> Switch19/3
  [VHAL_Flashdatatrust_flg] -> Switch19/2
  Constant23/1 -> Switch20/3
  [VHAL_Flashdatatrust_flg] -> Switch20/2
  Constant24/1 -> Switch21/3
  [VHAL_Flashdatatrust_flg] -> Switch21/2
  Constant25/1 -> Switch22/3
  [VHAL_Flashdatatrust_flg] -> Switch22/2
  [VHAL_LFPindi_enum] -> Switch19/1
  [VHAL_RFPindi_enum] -> Switch20/1
  [VHAL_LRPindi_enum] -> Switch21/1
  [VHAL_RRPindi_enum] -> Switch22/1
  Constant26/1 -> Switch23/3
  [VHAL_Flashdatatrust_flg] -> Switch23/2
  [VHAL_LFP20_raw8] -> Switch23/1
  Constant27/1 -> Switch24/3
  [VHAL_Flashdatatrust_flg] -> Switch24/2
  [VHAL_RFP20_raw8] -> Switch24/1
  Constant28/1 -> Switch25/3
  [VHAL_Flashdatatrust_flg] -> Switch25/2
  [VHAL_LRP20_raw8] -> Switch25/1
  Constant29/1 -> Switch26/3
  [VHAL_Flashdatatrust_flg] -> Switch26/2
  [VHAL_RRP20_raw8] -> Switch26/1
  Constant30/1 -> Switch27/3
  [VHAL_LFWheelPress_raw8] -> Switch27/1
  Constant31/1 -> Switch28/3
  [VHAL_RFWheelPress_raw8] -> Switch28/1
  Constant32/1 -> Switch29/3
  [VHAL_LRWheelPress_raw8] -> Switch29/1
  Constant33/1 -> Switch30/3
  [VHAL_RRWheelPress_raw8] -> Switch30/1
  Constant34/1 -> Switch31/3
  [VHAL_LFWheelTemp_C] -> Switch31/1
  Constant35/1 -> Switch32/3
  [VHAL_RFWheelTemp_C] -> Switch32/1
  Constant36/1 -> Switch33/3
  [VHAL_LRWheelTemp_C] -> Switch33/1
  Constant37/1 -> Switch34/3
  Logical Operator2/1 -> Switch34/2
  Constant38/1 -> Switch35/3
  [VHAL_unlearnSfali_flg] -> Switch35/1
  [VHAL_RRWheelTemp_C] -> Switch34/1
  Switch12/1 -> VHAL_FlashRFSensorFail_flg/1
  Switch13/1 -> VHAL_FlashLRSensorFail_flg/1
  Switch14/1 -> VHAL_FlashRRSensorFail_flg/1
  Switch15/1 -> VHAL_FlashLFWheelPSW_raw8/1
  Switch16/1 -> VHAL_FlashRFWheelPSW_raw8/1
  Switch17/1 -> VHAL_FlashLRWheelPSW_raw8/1
  Switch18/1 -> VHAL_FlashRRWheelPSW_raw8/1
  Switch19/1 -> VHAL_FlashLFPindi_enum/1
  Switch20/1 -> VHAL_FlashRFPindi_enum/1
  Switch21/1 -> VHAL_FlashLRPindi_enum/1
  Switch22/1 -> VHAL_FlashRRPindi_enum/1
  Switch23/1 -> VHAL_FlashLFP20_raw8/1
  Switch24/1 -> VHAL_FlashRFP20_raw8/1
  Switch25/1 -> VHAL_FlashLRP20_raw8/1
  Switch26/1 -> VHAL_FlashRRP20_raw8/1
  Switch27/1 -> VHAL_FlashLFWheelPress_raw8/1
  Switch28/1 -> VHAL_FlashRFWheelPress_raw8/1
  Switch29/1 -> VHAL_FlashLRWheelPress_raw8/1
  Switch30/1 -> VHAL_FlashRRWheelPress_raw8/1
  Switch31/1 -> VHAL_FlashLFWheelTemp_C/1
  Switch32/1 -> VHAL_FlashRFWheelTemp_C/1
  Switch33/1 -> VHAL_FlashLRWheelTemp_C/1
  Switch34/1 -> VHAL_FlashRRWheelTemp_C/1
  [VHAL_unlearnSfailvalid_enum] -> Relational Operator2/1
  Constant39/1 -> Relational Operator2/2
  Constant40/1 -> Switch36/1
  [VHAL_TPMSResButt_flg] -> Switch36/2
  Switch35/1 -> VHAL_FlashunlearnSfali_flg/1
  Switch36/1 -> Switch35/2
  Relational Operator2/1 -> Switch36/3
  Constant42/1 -> Relational Operator3/2
  [VHAL_TPMSResButt_flg] -> Switch37/2
  Constant41/1 -> Switch37/1
  Relational Operator3/1 -> Switch37/3
  [VHAL_Prepresstempvalid_enum] -> Relational Operator3/1
  Switch37/1 -> VHAL_Prepresstemptrust_flg/1, [VHAL_Prepresstemptrust_flg]
  [VHAL_Flashdatatrust_flg] -> Logical Operator2/1
  [VHAL_Prepresstemptrust_flg] -> Logical Operator2/2
  [VHAL_Flashdatatrust_flg] -> Logical Operator3/1
  [VHAL_Prepresstemptrust_flg] -> Logical Operator3/2
  Logical Operator3/1 -> Switch33/2
  [VHAL_Flashdatatrust_flg] -> Logical Operator4/1
  [VHAL_Prepresstemptrust_flg] -> Logical Operator4/2
  Logical Operator4/1 -> Switch32/2
  [VHAL_Flashdatatrust_flg] -> Logical Operator5/1
  [VHAL_Prepresstemptrust_flg] -> Logical Operator5/2
  Logical Operator5/1 -> Switch31/2
  [VHAL_Flashdatatrust_flg] -> Logical Operator6/1
  [VHAL_Prepresstemptrust_flg] -> Logical Operator6/2
  Logical Operator6/1 -> Switch30/2
  [VHAL_Flashdatatrust_flg] -> Logical Operator7/1
  [VHAL_Prepresstemptrust_flg] -> Logical Operator7/2
  Logical Operator7/1 -> Switch29/2
  [VHAL_Flashdatatrust_flg] -> Logical Operator8/1
  [VHAL_Prepresstemptrust_flg] -> Logical Operator8/2
  Logical Operator8/1 -> Switch28/2
  [VHAL_Flashdatatrust_flg] -> Logical Operator9/1
  [VHAL_Prepresstemptrust_flg] -> Logical Operator9/2
  Logical Operator9/1 -> Switch27/2
  Detect Increase/1 -> Latch/1
  Data Type Conversion/1 -> VHAL_LFID_raw/1
  Data Type Conversion1/1 -> VHAL_RFID_raw/1
  Data Type Conversion2/1 -> VHAL_LRID_raw/1
  Data Type Conversion3/1 -> VHAL_RRID_raw/1
  Data Type Conversion4/1 -> VHAL_ChkLFID_raw/1
  Data Type Conversion5/1 -> VHAL_ChkRFID_raw/1
  Data Type Conversion6/1 -> VHAL_ChkLRID_raw/1
  Data Type Conversion7/1 -> VHAL_ChkRRID_raw/1
  Switch42/1 -> [VHAL_FlashIDtrust_flg]
  Constant45/1 -> Switch40/3
  Constant46/1 -> Switch41/3
  Constant44/1 -> Switch39/3
  Switch39/1 -> VHAL_S2ID_raw/1
  [VHAL_FlashS3ID_raw] -> Switch40/1
  [VHAL_FlashS2ID_raw] -> Switch39/1
  [VHAL_FlashS4ID_raw] -> Switch41/1
  Constant43/1 -> Switch38/3
  [VHAL_FlashS1ID_raw] -> Switch38/1
  [VHAL_TPMSResButt_flg] -> Switch42/2
  [VHAL_FlashIDtrust_flg] -> Switch38/2
  Switch41/1 -> VHAL_S4ID_raw/1
  [VHAL_FlashIDtrust_flg] -> Switch39/2
  Constant47/1 -> Switch42/1
  Switch40/1 -> VHAL_S3ID_raw/1
  Constant48/1 -> Relational Operator4/2
  [VHAL_FlashIDtrust_flg] -> Switch41/2
  Switch38/1 -> VHAL_S1ID_raw/1
  [VHAL_FlashIDvalid_enum] -> Relational Operator4/1
  Relational Operator4/1 -> Switch42/3
  [VHAL_FlashIDtrust_flg] -> Switch40/2
  Bus Selector1/35 -> [VHAL_unlearnSfali_flg]  "<VHAL_unlearnSfali_flg>"
  Bus Selector1/4 -> [VHAL_FlashChkRRID]  "<VHAL_FlashChkRRID_raw>"
  Bus Selector1/27 -> [VHAL_LFWheelPress_raw8]  "<VHAL_LFWheelPress_raw8>"
  Bus Selector1/19 -> [VHAL_LFPindi_enum]  "<VHAL_LFPindi_enum>"
  Bus Selector1/21 -> [VHAL_LRPindi_enum]  "<VHAL_LRPindi_enum>"
  Bus Selector1/25 -> [VHAL_LRP20_raw8]  "<VHAL_LRP20_raw8>"
  Bus Selector1/33 -> [VHAL_LRWheelTemp_C]  "<VHAL_LRWheelTemp_C>"
  Bus Selector1/26 -> [VHAL_RRP20_raw8]  "<VHAL_RRP20_raw8>"
  Bus Selector1/18 -> [VHAL_RRWheelPSW_raw8]  "<VHAL_RRWheelPSW_raw8>"
  Bus Selector1/32 -> [VHAL_RFWheelTemp_C]  "<VHAL_RFWheelTemp_C>"
  Bus Selector1/29 -> [VHAL_LRWheelPress_raw8]  "<VHAL_LRWheelPress_raw8>"
  Bus Selector1/8 -> [VHAL_FlashRRID]  "<VHAL_FlashRRID_raw>"
  Bus Selector1/12 -> [VHAL_RFSensorFail_flg]  "<VHAL_RFSensorFail_flg>"
  Bus Selector1/20 -> [VHAL_RFPindi_enum]  "<VHAL_RFPindi_enum>"
  Bus Selector1/11 -> [VHAL_LFSensorFail_flg]  "<VHAL_LFSensorFail_flg>"
  Bus Selector1/24 -> [VHAL_RFP20_raw8]  "<VHAL_RFP20_raw8>"
  Bus Selector1/22 -> [VHAL_RRPindi_enum]  "<VHAL_RRPindi_enum>"
  Bus Selector1/6 -> [VHAL_FlashRFID]  "<VHAL_FlashRFID_raw>"
  Bus Selector1/3 -> [VHAL_FlashChkLRID]  "<VHAL_FlashChkLRID_raw>"
  Bus Selector1/2 -> [VHAL_FlashChkRFID]  "<VHAL_FlashChkRFID_raw>"
  Bus Selector1/37 -> [VHAL_Prepresstempvalid_enum]  "<VHAL_Prepresstempvalid_enum>"
  Bus Selector1/34 -> [VHAL_RRWheelTemp_C]  "<VHAL_RRWheelTemp_C>"
  Bus Selector1/16 -> [VHAL_RFWheelPSW_raw8]  "<VHAL_RFWheelPSW_raw8>"
  Bus Selector1/30 -> [VHAL_RRWheelPress_raw8]  "<VHAL_RRWheelPress_raw8>"
  Bus Selector1/28 -> [VHAL_RFWheelPress_raw8]  "<VHAL_RFWheelPress_raw8>"
  Bus Selector1/14 -> [VHAL_RRSensorFail_flg]  "<VHAL_RRSensorFail_flg>"
  Bus Selector1/38 -> [VHAL_FlashS1ID_raw]  "<VHAL_FlashS1ID_raw>"
  Bus Selector1/41 -> [VHAL_FlashS4ID_raw]  "<VHAL_FlashS4ID_raw>"
  Bus Selector1/10 -> [VHAL_Flashdatavalid_enum]  "<VHAL_Flashdatavalid_enum>"
  Bus Selector1/15 -> [VHAL_LFWheelPSW_raw8]  "<VHAL_LFWheelPSW_raw8>"
  Bus Selector1/5 -> [VHAL_FlashLFID]  "<VHAL_FlashLFID_raw>"
  Bus Selector1/39 -> [VHAL_FlashS2ID_raw]  "<VHAL_FlashS2ID_raw>"
  BHAL_SYSTPMS_outputs/1 -> Bus Selector1/1
  Bus Selector1/9 -> [VHAL_Flashchkdatavalid_enum]  "<VHAL_Flashchkdatavalid_enum>"
  Bus Selector1/1 -> [VHAL_FlashChkLFID]  "<VHAL_FlashChkLFID_raw>"
  Bus Selector1/7 -> [VHAL_FlashLRID]  "<VHAL_FlashLRID_raw>"
  Bus Selector1/36 -> [VHAL_unlearnSfailvalid_enum]  "<VHAL_unlearnSfailvalid_enum>"
  Bus Selector1/23 -> [VHAL_LFP20_raw8]  "<VHAL_LFP20_raw8>"
  Bus Selector1/40 -> [VHAL_FlashS3ID_raw]  "<VHAL_FlashS3ID_raw>"
  Bus Selector1/13 -> [VHAL_LRSensorFail_flg]  "<VHAL_LRSensorFail_flg>"
  Bus Selector1/42 -> [VHAL_FlashIDvalid_enum]  "<VHAL_FlashIDvalid_enum>"
  Bus Selector1/31 -> [VHAL_LFWheelTemp_C]  "<VHAL_LFWheelTemp_C>"
  Bus Selector1/17 -> [VHAL_LRWheelPSW_raw8]  "<VHAL_LRWheelPSW_raw8>"
  Bus Selector1/43 -> Data Type Conversion8/1  "<VHAL_TPMSSensorIDRegSta_raw>"
  [VHAL_TPMSSensorIDRegSta_enum] -> VHAL_TPMSSensorIDRegSta_enum/1
  Data Type Conversion8/1 -> [VHAL_TPMSSensorIDRegSta_enum]  "VHAL_TPMSSensorIDRegSta_enum"
